simulink model "ysw12_2"  (R2014a)
settings: Solver=ode45  StartTime=0.0  StopTime=300  RelTol=1e-3
undefined symbols (not defined in the file or in its folder): BP_PID
settings Model: Creator=Administrator  LastModifiedBy=Administrator

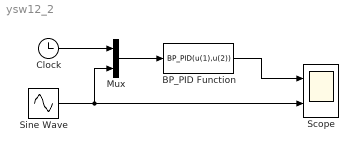
== system ysw12_2 ==
  BP_PID Function : MATLABFcn  MATLABFcn=BP_PID(u(1),u(2))
  Clock : Clock
  Mux : Mux  Inputs=2
  Scope : Scope  NumInputPorts=2
      settings: YMin=-5~-5  YMax=5~5
  Sine Wave : Sin  Frequency=2*pi*2*0.001  SampleTime=0
  wires:
  Mux/1 -> BP_PID Function/1
  BP_PID Function/1 -> Scope/1
  Clock/1 -> Mux/1
  Sine Wave/1 -> Mux/2, Scope/2
